simulink model "LGR_FM"  (R2014a)
settings: Solver=ode45  StartTime=0.0  StopTime=600  RelTol=1e-3
values from neighbouring files (symbols this model uses):
  DenC1_LGR = [1 0]    [ControladorDescentralizadoLGReIMC.m]    (also in FNM_ControladorDescentralizadoLGReIMC.m = [1 0 0 0])
  DenC2_LGR = [1 0]    [ControladorDescentralizadoLGReIMC.m]    (also in FNM_ControladorDescentralizadoLGReIMC.m = [1 0 0 0])
  NumC1_LGR = [KK1 KK1*Zc1]    [ControladorDescentralizadoLGReIMC.m]    (also in FNM_ControladorDescentralizadoLGReIMC.m)
  NumC2_LGR = [KK2 KK2*Zc2]    [ControladorDescentralizadoLGReIMC.m]    (also in FNM_ControladorDescentralizadoLGReIMC.m)
settings Model: Creator=Imaculada  LastModifiedBy=Imaculada

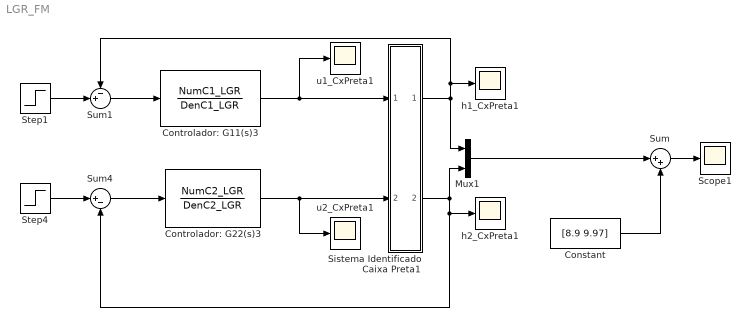
== system LGR_FM ==
  Constant : Constant  Value=[8.9 9.97]
  Controlador: G11(s)3 : TransferFcn  Numerator=NumC1_LGR  Denominator=DenC1_LGR
  Controlador: G22(s)3 : TransferFcn  Numerator=NumC2_LGR  Denominator=DenC2_LGR
  Mux1 : Mux  Inputs=2
  Scope1 : Scope
      settings: SaveName=Simulado
  Sistema Identificado Caixa Preta1 : Subsystem
  Step1 : Step  Time=200  SampleTime=0
  Step4 : Step  Time=500  SampleTime=0
  Sum : Sum  Inputs=|++
  Sum1 : Sum  Inputs=-+|
  Sum4 : Sum  Inputs=|+-
  h1_CxPreta1 : Scope
      settings: SaveName=ScopeData6
  h2_CxPreta1 : Scope
      settings: SaveName=ScopeData7
  u1_CxPreta1 : Scope
      settings: SaveName=ScopeData8
  u2_CxPreta1 : Scope
      settings: SaveName=ScopeData9
  wires:
  Sistema Identificado Caixa Preta1/1(h1) -> Mux1/1, Sum1/1, h1_CxPreta1/1
  Sistema Identificado Caixa Preta1/2(h2) -> h2_CxPreta1/1, Sum4/2, Mux1/2
  Controlador: G22(s)3/1 -> Sistema Identificado Caixa Preta1/2(u2), u2_CxPreta1/1
  Step1/1 -> Sum1/2
  Step4/1 -> Sum4/1
  Controlador: G11(s)3/1 -> Sistema Identificado Caixa Preta1/1(u1), u1_CxPreta1/1
  Sum1/1 -> Controlador: G11(s)3/1
  Sum4/1 -> Controlador: G22(s)3/1
  Sum/1 -> Scope1/1
  Mux1/1 -> Sum/1
  Constant/1 -> Sum/2

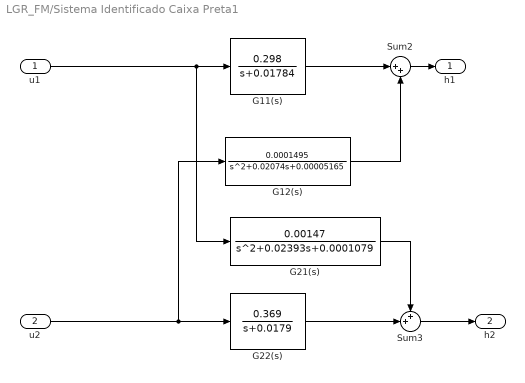
== system LGR_FM/Sistema Identificado Caixa Preta1 ==
  u1 : Inport
  u2 : Inport  Port=2
  G11(s) : TransferFcn  Numerator=[0 0.298]  Denominator=[1 0.01784]
  G12(s) : TransferFcn  Numerator=[0 0 0.0001495]  Denominator=[1 0.02074 0.00005165]
  G21(s) : TransferFcn  Numerator=[0 0 0.00147]  Denominator=[1 0.02393 0.0001079]
  G22(s) : TransferFcn  Numerator=[0 0.369]  Denominator=[1 0.0179]
  Sum2 : Sum  Inputs=|++
  Sum3 : Sum  Inputs=++|
  h1 : Outport
  h2 : Outport  Port=2
  wires:
  G11(s)/1 -> Sum2/1
  G22(s)/1 -> Sum3/2
  G12(s)/1 -> Sum2/2
  G21(s)/1 -> Sum3/1
  Sum2/1 -> h1/1
  Sum3/1 -> h2/1
  u1/1 -> G21(s)/1, G11(s)/1
  u2/1 -> G12(s)/1, G22(s)/1
